simulink model "aero_radmod"  (R2019b)
settings: Solver=ode5  StartTime=0.0  StopTime=100  FixedStep=0.1  MaxStep=0.1  RelTol=1e-3  AbsTol=1e-6
StopFcn:
  | aero_radplot;
undefined symbols (not defined in the file): deltat, g, tauc, tauT
libraries: simulink x2
CloseFcn:
  | h=findobj('type','figure');if ~isempty(h);close(h);end
settings Model: ExtModeTrigMode=oneshot  ExtModeArmWhenConnect=off  ExtModeAutoUpdateStatusClock=off  Creator=The MathWorks Inc.  LastModifiedBy=Nikhil
settings SolverCC: AutoScaleAbsTol=off
settings DataIOCC: SaveFormat=Array  SignalLoggingSaveFormat=ModelDataLogs  SaveOutput=off  ReturnWorkspaceOutputs=off  TimeSaveName=t_sim
settings OptimizationCC: BlockReduction=off  BooleanDataType=off  ExpressionDepthLimit=2147483647  InitFltsAndDblsToZero=on  LifeSpan=inf
settings DebuggingCC: SaveWithParameterizedLinksMsg=none  UnderspecifiedInitializationDetection=Classic  MergeDetectMultiDrivingBlocksExec=none  SignalResolutionControl=TryResolveAllWithWarning  MultiTaskDSMMsg=warning  MultiTaskCondExecSysMsg=none  FcnCallInpInsideContextMsg=warning  StateNameClashWarn=warning  SFUnexpectedBacktrackingDiag=warning  SFNoUnconditionalDefaultTransitionDiag=warning  SFExecutionAtInitializationDiag=none  ArithmeticOperatorsInVariantConditions=warning
settings HardwareCC: ProdBitPerPointer=32  ProdBitPerSizeT=32  ProdBitPerPtrDiffT=32  ProdLargestAtomicFloat=None  ProdIntDivRoundTo=Undefined  ProdEndianess=Unspecified  ProdWordSize=32  ProdHWDeviceType=32-bit Generic  TargetUnknown=on
settings ModelReferenceCC: EnableRefExpFcnMdlSchedulingChecks=off  PropagateSignalLabelsOutOfModel=off
settings RTWCC: Description=Generic Real-Time Target  MakeCommand="make_rtw  OPTS=-D"  TemplateMakefile=grt_vc.tmf
settings CodeAppCC: StateflowObjectComments=on
settings GRTTargetCC: TargetFcnLib=ansi_tfl_tmw.mat  TargetLangStandard=C89/C90 (ANSI)  CombineOutputUpdateFcns=off  GRTInterface=on
settings ConfigComp: CovMetricSettings=d  CovSaveCumulativeToWorkspaceVar=on  CovSaveSingleToWorkspaceVar=on

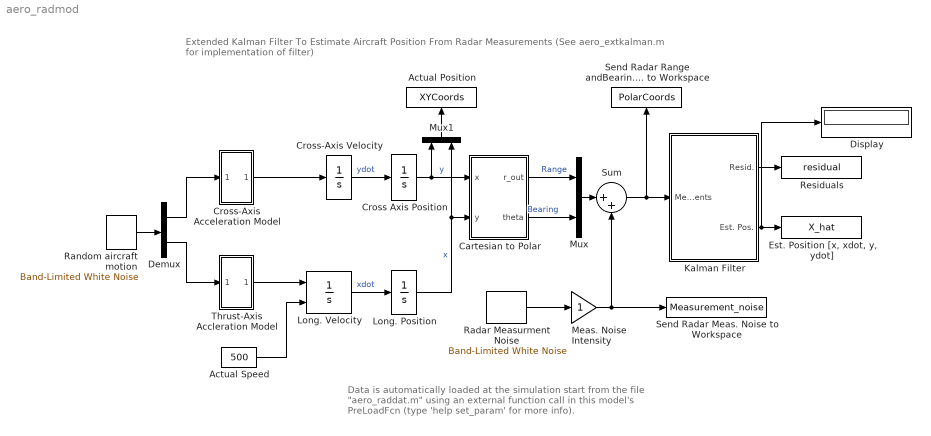
== system aero_radmod ==
  note: Data is automatically loaded at the simulation start from the file
      | "aero_raddat.m"
      | using an external function call in this model's PreLoadFcn
      | (type 'help set_param' for more info).
  note: Extended Kalman Filter To Estimate Aircraft Position From Radar Measurements
      | (See aero_extkalman.m for implementation of filter)
  Actual Position : ToWorkspace  VariableName=XYCoords
  Actual Speed : Constant  Value=500
  Cartesian to Polar : Subsystem  mask([x,y]->[r,theta]){}
      mask help:
      | Tranformation from cartesian to polar
      | coordinates.
      | r=sqrt(x^2+y^2), theta=atan(y/x)
      mask Help: Unmask this block for more help.
      mask Display: plot(0,0,100,100,[24,20,15,20,20],[85,95,85,95,20],[80,20,95,85,95,85],[70,20,20,15,20,24],[56,56,55,52,50,46],[20,26,31,35,38,42])
  "Cross Axis Position " : Integrator
  Cross-Axis Acceleration Model : Subsystem
  Cross-Axis Velocity : Integrator
  Demux : Demux  Outputs=2
  Display : Display
  "Est. Position [x, xdot, y, ydot]" : ToWorkspace  VariableName=X_hat  SampleTime=-1
  Kalman Filter : Subsystem
  Long. Position : Integrator
  Long. Velocity : Integrator  InitialConditionSource=external
  Meas. Noise Intensity : Gain  SaturateOnIntegerOverflow=on  OutDataTypeStr=Inherit: Same as input  ParamDataTypeStr=Inherit: Same as input
  Mux : Mux  Inputs=2
  Mux1 : Mux  Inputs=2
  Radar Measurment Noise : simulink/Sources/Band-Limited White Noise  Cov=[1 1]  Ts=0.1  seed=[52341 62341]
  Random aircraft motion : simulink/Sources/Band-Limited White Noise  Cov=[0.001 .001]  Ts=0.1  seed=[58413 74925]
  Residuals : ToWorkspace  VariableName=residual  SampleTime=-1
  Send Radar Meas. Noise to Workspace : ToWorkspace  VariableName=Measurement_noise
  Send Radar Range andBearing Angle Meas. to Workspace : ToWorkspace  VariableName=PolarCoords  SampleTime=-1
  Sum : Sum  Inputs=|++  SaturateOnIntegerOverflow=on  InputSameDT=on  OutDataTypeStr=Inherit: Same as first input
  Thrust-Axis Accleration Model : Subsystem
  wires:
  Long. Position/1 -> Mux1/2, Cartesian to Polar/2(y)  "x"
  Cartesian to Polar/2(theta) -> Mux/2  "Bearing"
  Cartesian to Polar/1(r_out) -> Mux/1  "Range"
  Mux/1 -> Sum/1
  Sum/1 -> Kalman Filter/1(Measurements), Send Radar Range andBearing Angle Meas. to Workspace/1
  "Cross Axis Position "/1 -> Mux1/1, Cartesian to Polar/1(x)  "y"
  Cross-Axis Acceleration Model/1(out_1) -> Cross-Axis Velocity/1
  Cross-Axis Velocity/1 -> "Cross Axis Position "/1  "ydot"
  Actual Speed/1 -> Long. Velocity/2
  Long. Velocity/1 -> Long. Position/1  "xdot"
  Thrust-Axis Accleration Model/1(Accleration) -> Long. Velocity/1
  Kalman Filter/1(Resid.) -> Residuals/1
  Demux/1 -> Cross-Axis Acceleration Model/1(Inport)
  Demux/2 -> Thrust-Axis Accleration Model/1(Force)
  Random aircraft motion/1 -> Demux/1
  Kalman Filter/2(Est. Pos.) -> "Est. Position [x, xdot, y, ydot]"/1, Display/1
  Mux1/1 -> Actual Position/1
  Radar Measurment Noise/1 -> Meas. Noise Intensity/1
  Meas. Noise Intensity/1 -> Send Radar Meas. Noise to Workspace/1, Sum/2

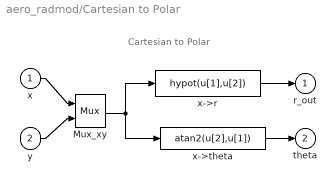
== system aero_radmod/Cartesian to Polar ==
  note: Cartesian to Polar
  x : Inport
  y : Inport  Port=2
  Mux_xy : Mux  Inputs=2
  x->r : Fcn  Expr=hypot(u[1],u[2])
  x->theta : Fcn  Expr=atan2(u[2],u[1])
  r_out : Outport
  theta : Outport  Port=2
  wires:
  Mux_xy/1 -> x->r/1, x->theta/1
  x->r/1 -> r_out/1
  x/1 -> Mux_xy/1
  y/1 -> Mux_xy/2
  x->theta/1 -> theta/1

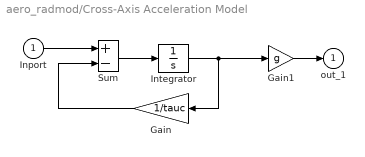
== system aero_radmod/Cross-Axis Acceleration Model ==
  Inport : Inport
  Gain : Gain  Gain=1/tauc  SaturateOnIntegerOverflow=on  OutDataTypeStr=Inherit: Same as input  ParamDataTypeStr=Inherit: Same as input
  Gain1 : Gain  Gain=g  SaturateOnIntegerOverflow=on  OutDataTypeStr=Inherit: Same as input  ParamDataTypeStr=Inherit: Same as input
  Integrator : Integrator
  Sum : Sum  Inputs=+-  SaturateOnIntegerOverflow=on  InputSameDT=on  OutDataTypeStr=Inherit: Same as first input
  out_1 : Outport
  wires:
  Inport/1 -> Sum/1
  Gain/1 -> Sum/2
  Integrator/1 -> Gain1/1, Gain/1
  Sum/1 -> Integrator/1
  Gain1/1 -> out_1/1

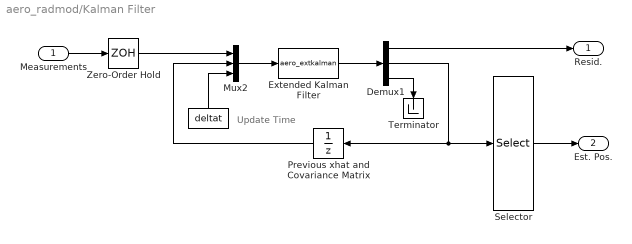
== system aero_radmod/Kalman Filter ==
  note: Update Time
  Measurements : Inport
  " " : Constant  Value=deltat
  Demux1 : Demux  Outputs=[2 20 1]
  Extended Kalman Filter : MATLABFcn  MATLABFcn=aero_extkalman  OutputDimensions=23
  Mux2 : Mux  Inputs=3
  Previous xhat and Covariance Matrix : UnitDelay  InitialCondition=[0.001; 0.01; 0.001; 400; zeros(16,1)]  SampleTime=deltat
  Selector : Selector  InputPortWidth=20  IndexOptions=Index vector (dialog)  Indices=[1:4]  OutputSizes=1
  Terminator : Terminator
  Zero-Order Hold : ZeroOrderHold  SampleTime=deltat
  Resid. : Outport
  Est. Pos. : Outport  Port=2
  wires:
  Measurements/1 -> Zero-Order Hold/1
  Extended Kalman Filter/1 -> Demux1/1
  Zero-Order Hold/1 -> Mux2/1
  Selector/1 -> Est. Pos./1
  Demux1/1 -> Resid./1
  Demux1/2 -> Previous xhat and Covariance Matrix/1, Selector/1
  " "/1 -> Mux2/3
  Previous xhat and Covariance Matrix/1 -> Mux2/2
  Mux2/1 -> Extended Kalman Filter/1
  Demux1/3 -> Terminator/1

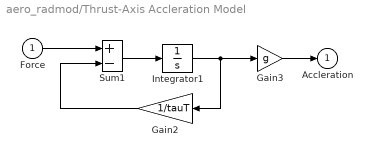
== system aero_radmod/Thrust-Axis Accleration Model ==
  Force : Inport
  Gain2 : Gain  Gain=1/tauT  SaturateOnIntegerOverflow=on  OutDataTypeStr=Inherit: Same as input  ParamDataTypeStr=Inherit: Same as input
  Gain3 : Gain  Gain=g  SaturateOnIntegerOverflow=on  OutDataTypeStr=Inherit: Same as input  ParamDataTypeStr=Inherit: Same as input
  Integrator1 : Integrator
  Sum1 : Sum  Inputs=+-  SaturateOnIntegerOverflow=on  InputSameDT=on  OutDataTypeStr=Inherit: Same as first input
  Accleration : Outport
  wires:
  Force/1 -> Sum1/1
  Gain2/1 -> Sum1/2
  Integrator1/1 -> Gain3/1, Gain2/1
  Sum1/1 -> Integrator1/1
  Gain3/1 -> Accleration/1
